simulink model "practice4"  (R2014a)
settings: Solver=VariableStepDiscrete  StartTime=0.0  StopTime=100  RelTol=1e-3
settings Model: Creator=Huanglei  LastModifiedBy=Huanglei

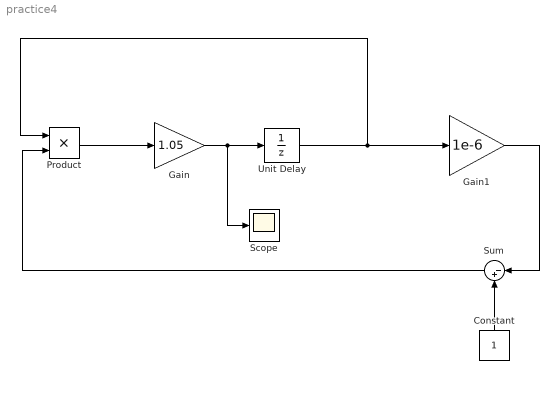
== system practice4 ==
  Constant : Constant
  Gain : Gain  Gain=1.05
  Gain1 : Gain  Gain=1e-6
  Product : Product
  Scope : Scope
  Sum : Sum  Inputs=|-+
  Unit Delay : UnitDelay  InitialCondition=100000
  wires:
  Product/1 -> Gain/1
  Gain/1 -> Scope/1, Unit Delay/1
  Unit Delay/1 -> Product/1, Gain1/1
  Gain1/1 -> Sum/1
  Constant/1 -> Sum/2
  Sum/1 -> Product/2
